simulink model "PC4_DCS_810698349"  (R2021b)
settings: Solver=VariableStepAuto  StartTime=0.0  StopTime=3  RelTol=1e-3
undefined symbols (not defined in the file): C, G, H, Kc, Lo, N, Ts, y0, y00
libraries: simulink x1
settings Model: Creator=SinaK  LastModifiedBy=SinaK

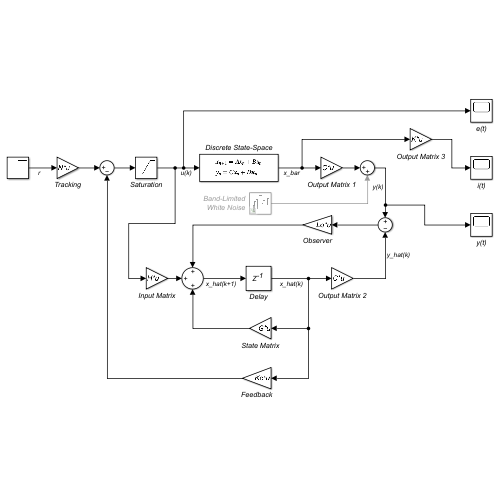
[thumbnail: Simulink's stored preview of the top-level diagram]
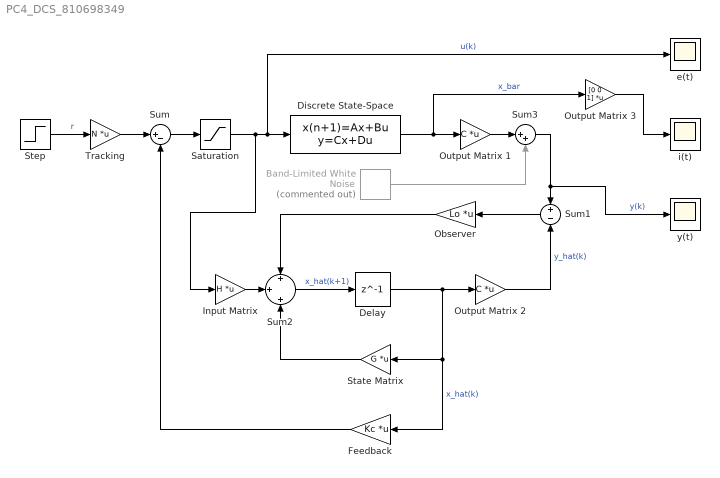
== system PC4_DCS_810698349 ==
  Band-Limited White Noise : simulink/Sources/Band-Limited White Noise  Commented=on  Cov=[0.000001]*y0*y0  Ts=Ts*10  seed=[23341]
  Delay : Delay  DelayLength=1  SampleTime=Ts
  Discrete State-Space : DiscreteStateSpace  A=G  B=H  C=eye(3)  D=[0;0;0]  InitialCondition=[y00 0 0]  SampleTime=Ts
  Feedback : Gain  Gain=Kc  Multiplication=Matrix(K*u)
  Input Matrix : Gain  Gain=H  Multiplication=Matrix(K*u)
  Observer : Gain  Gain=Lo  Multiplication=Matrix(K*u)
  Output Matrix 1 : Gain  Gain=C  Multiplication=Matrix(K*u)
  Output Matrix 2 : Gain  Gain=C  Multiplication=Matrix(K*u)
  Output Matrix 3 : Gain  Gain=[0 0 1]  Multiplication=Matrix(K*u)
  Saturation : Saturate  UpperLimit=12  LowerLimit=0
  State Matrix : Gain  Gain=G  Multiplication=Matrix(K*u)
  Step : Step  Time=0  After=y0  SampleTime=Ts
  Sum : Sum  Inputs=|+-
  Sum1 : Sum  Inputs=+|-
  Sum2 : Sum  Inputs=+|+|+
  Sum3 : Sum  Inputs=|++
  Tracking : Gain  Gain=N  Multiplication=Matrix(K*u)
  e(t) : Scope
  i(t) : Scope
  y(t) : Scope
  wires:
  Tracking/1 -> Sum/1
  Sum1/1 -> Observer/1
  Observer/1 -> Sum2/1
  Input Matrix/1 -> Sum2/2
  State Matrix/1 -> Sum2/3
  Sum2/1 -> Delay/1  "x_hat(k+1)"
  Delay/1 -> Output Matrix 2/1, Feedback/1, State Matrix/1  "x_hat(k)"
  Output Matrix 2/1 -> Sum1/2  "y_hat(k)"
  Feedback/1 -> Sum/2
  Discrete State-Space/1 -> Output Matrix 3/1, Output Matrix 1/1  "x_bar"
  Sum/1 -> Saturation/1
  Saturation/1 -> Input Matrix/1, e(t)/1, Discrete State-Space/1  "u(k)"
  Output Matrix 3/1 -> i(t)/1
  Step/1 -> Tracking/1  "r"
  Output Matrix 1/1 -> Sum3/1
  Sum3/1 -> y(t)/1, Sum1/1  "y(k)"
  Band-Limited White Noise/1 -> Sum3/2
